simulink subsystem "Pump"  (R2019b)
settings: Solver=VariableStepAuto  StartTime=0.0  StopTime=10.0  RelTol=1e-3
values from neighbouring files (symbols this model uses):
  k11 = k2^2+4*(k-k3)*k1    (= 0.0933546)    [part1.m]
  k12 = 8*(k-k3)    (= 0.2848)    [part1.m]
  k13 = 2*(k-k3)    (= 0.0712)    [part1.m]
  k2 = -0.015    [part1.m]
settings Model: Creator=ovi  LastModifiedBy=ovi

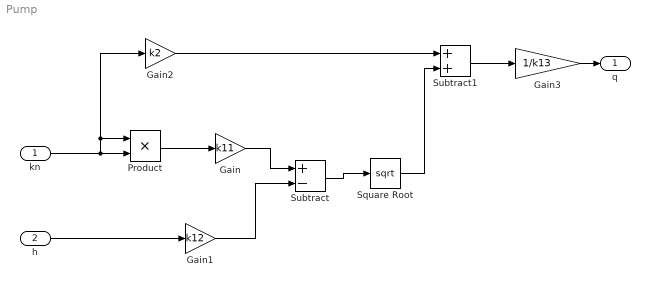
== system Pump ==
  kn : Inport
  h : Inport  Port=2
  Gain : Gain  Gain=k11
  Gain1 : Gain  Gain=k12
  Gain2 : Gain  Gain=k2
  Gain3 : Gain  Gain=1/k13
  Product : Product
  Square Root : Sqrt  SaturateOnIntegerOverflow=on
  Subtract : Sum  Inputs=+-
  Subtract1 : Sum
  q : Outport
  wires:
  kn/1 -> Gain2/1, Product/1, Product/2
  Product/1 -> Gain/1
  h/1 -> Gain1/1
  Gain1/1 -> Subtract/2
  Gain/1 -> Subtract/1
  Subtract/1 -> Square Root/1
  Gain2/1 -> Subtract1/1
  Square Root/1 -> Subtract1/2
  Subtract1/1 -> Gain3/1
  Gain3/1 -> q/1
